simulink model "old_sync_block"  (R2015b)
settings: Solver=VariableStepAuto  StartTime=0.0  StopTime=10.0  RelTol=1e-3
undefined symbols (not defined in the file or in its folder): DiscIntNeverNeededParam, zh_step
libraries: simulink x2, dspnetwork x1
settings Model: Creator=Anony  LastModifiedBy=Anony

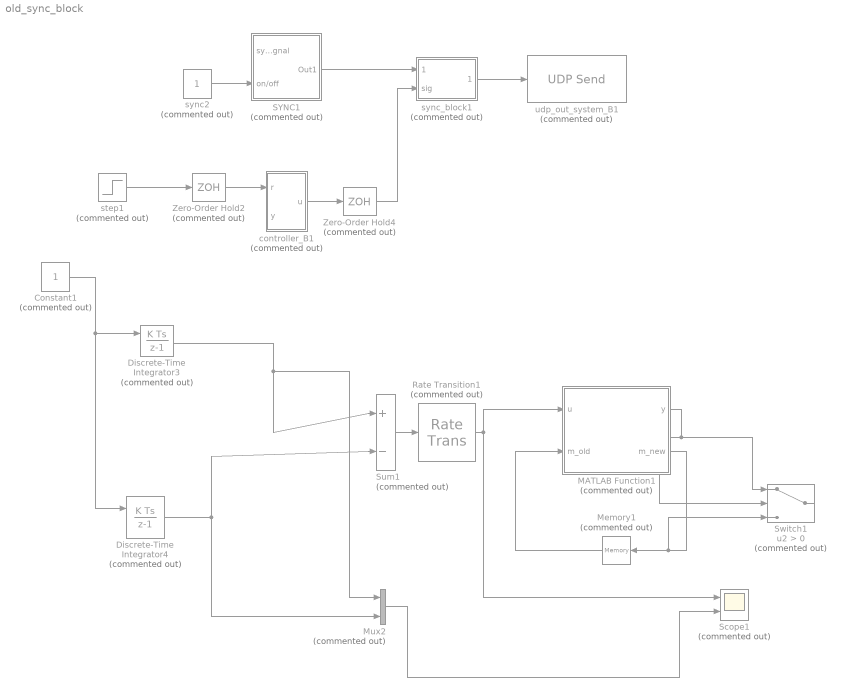
== system old_sync_block ==
  Constant1 : Constant  Commented=on
  Discrete-Time Integrator3 : DiscreteIntegrator  Commented=on  ExternalReset=rising  InitialConditionSetting=State (most efficient)  SampleTime=0.001  ICPrevOutput=DiscIntNeverNeededParam  ICPrevScaledInput=DiscIntNeverNeededParam
  Discrete-Time Integrator4 : DiscreteIntegrator  Commented=on  ExternalReset=rising  InitialConditionSetting=State (most efficient)  SampleTime=0.001  ICPrevOutput=DiscIntNeverNeededParam  ICPrevScaledInput=DiscIntNeverNeededParam
  MATLAB Function1 : MATLAB Function  Commented=on  TreatAsAtomicUnit=on
  Memory1 : Memory  Commented=on
  Mux2 : Mux  Commented=on  Inputs=2
  Rate Transition1 : RateTransition  Commented=on  OutPortSampleTimeOpt=Inherit
  SYNC1 : Subsystem  Commented=on
  Scope1 : Scope  Commented=on  NumInputPorts=2
  Sum1 : Sum  Commented=on  Inputs=|+-
  Switch1 : Switch  Commented=on  Criteria=u2 > Threshold
  Zero-Order Hold2 : ZeroOrderHold  Commented=on  SampleTime=zh_step
  Zero-Order Hold4 : ZeroOrderHold  Commented=on  SampleTime=zh_step
  controller_B1 : Subsystem  Commented=on
  step1 : Step  Commented=on  After=0.15  SampleTime=0
  sync2 : Constant  Commented=on
  sync_block1 : Subsystem  Commented=on
  udp_out_system_B1 : dspnetwork/UDP Send  Commented=on  remoteURL='129.10.131.51'  remotePort=27510  localURL='0.0.0.0'  localPortSource=Automatically determine  localPort=27000  sampletime=-1  separateLengthPort=0
  wires:
  step1/1 -> Zero-Order Hold2/1
  Zero-Order Hold2/1 -> controller_B1/1(r)
  controller_B1/1(u) -> Zero-Order Hold4/1
  sync_block1/1(sig out) -> udp_out_system_B1/1
  SYNC1/1(Out1) -> sync_block1/1(sync_sig)
  sync2/1 -> SYNC1/2(on/off)
  Zero-Order Hold4/1 -> sync_block1/2(sig)
  Discrete-Time Integrator3/1 -> Sum1/1, Mux2/1
  Constant1/1 -> Discrete-Time Integrator3/1, Discrete-Time Integrator4/1
  MATLAB Function1/2(m_new) -> Switch1/3, Memory1/1
  Sum1/1 -> Rate Transition1/1
  Memory1/1 -> MATLAB Function1/2(m_old)
  Discrete-Time Integrator4/1 -> Sum1/2, Mux2/2
  Mux2/1 -> Scope1/2
  MATLAB Function1/1(y) -> Switch1/1, Switch1/2
  Rate Transition1/1 -> MATLAB Function1/1(u), Scope1/1

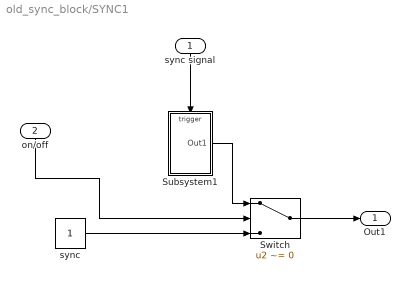
== system old_sync_block/SYNC1 ==
  sync signal : Inport
  on/off : Inport  Port=2
  Subsystem1 : Subsystem
  Switch : Switch  Criteria=u2 ~= 0
  sync : Constant
  Out1 : Outport
  wires:
  on/off/1 -> Switch/2
  Switch/1 -> Out1/1
  Subsystem1/1(Out1) -> Switch/1
  sync signal/1 -> Subsystem1/Trigger
  sync/1 -> Switch/3

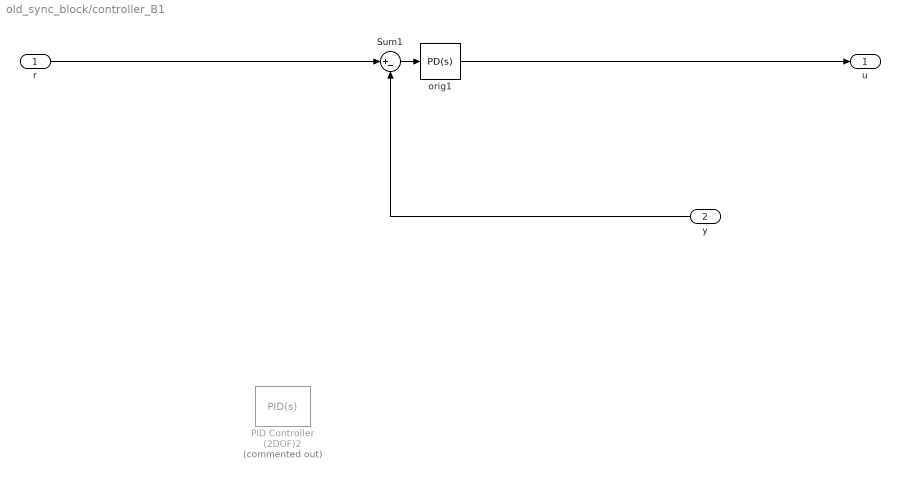
== system old_sync_block/controller_B1 ==
  r : Inport
  y : Inport  Port=2
  PID Controller (2DOF)2 : simulink/Continuous/PID Controller (2DOF)  Commented=on  Controller=PID  TimeDomain=Continuous-time  SampleTime=-1  IntegratorMethod=Forward Euler  FilterMethod=Forward Euler  Form=Parallel  UseFilter=on  ControllerParametersSource=internal  P=6.3799380872686  I=2.12979603411331  D=3.6093223618413  N=48.5068620404972  b=2.39624043732871  c=0.716079145801974  InitialConditionSource=internal  InitialConditionForIntegrator=0  InitialConditionForFilter=0  ExternalReset=none  LimitOutput=off  UpperSaturationLimit=inf  LowerSaturationLimit=-inf  LinearizeAsGain=on  AntiWindupMode=none  Kb=1  TrackingMode=off  Kt=1  PParamMin=[]  PParamMax=[]  IParamMin=[]  IParamMax=[]  DParamMin=[]  DParamMax=[]  NParamMin=[]  NParamMax=[]  bParamMin=[]  bParamMax=[]  cParamMin=[]  cParamMax=[]  KbParamMin=[]  KbParamMax=[]  KtParamMin=[]  KtParamMax=[]  POutMin=[]  POutMax=[]  IOutMin=[]  IOutMax=[]  DOutMin=[]  DOutMax=[]  NOutMin=[]  NOutMax=[]  bOutMin=[]  bOutMax=[]  cOutMin=[]  cOutMax=[]  KbOutMin=[]  KbOutMax=[]  KtOutMin=[]  KtOutMax=[]  IntegratorOutMin=[]  IntegratorOutMax=[]  FilterOutMin=[]  FilterOutMax=[]  SumOutMin=[]  SumOutMax=[]  Sum1OutMin=[]  Sum1OutMax=[]  Sum2OutMin=[]  Sum2OutMax=[]  Sum3OutMin=[]  Sum3OutMax=[]  SumI1OutMin=[]  SumI1OutMax=[]  SumI2OutMin=[]  SumI2OutMax=[]  SumI3OutMin=[]  SumI3OutMax=[]  SumDOutMin=[]  SumDOutMax=[]  SaturationOutMin=[]  SaturationOutMax=[]  IntegratorContinuousStateAttributes=''  IntegratorStateMustResolveToSignalObject=off  IntegratorRTWStateStorageClass=Auto  FilterContinuousStateAttributes=''  FilterStateMustResolveToSignalObject=off  FilterRTWStateStorageClass=Auto  DifferentiatorICPrevScaledInput=0  DifferentiatorOutMin=[]  DifferentiatorOutMax=[]
  Sum1 : Sum  Inputs=|+-
  orig1 : simulink/Continuous/PID Controller  Controller=PD  TimeDomain=Continuous-time  SampleTime=-1  IntegratorMethod=Forward Euler  FilterMethod=Forward Euler  Form=Parallel  UseFilter=on  ControllerParametersSource=internal  P=0.0142  I=0.0175856984919557  D=0.0001  N=100  InitialConditionSource=internal  InitialConditionForIntegrator=0  InitialConditionForFilter=0  ExternalReset=none  LimitOutput=on  UpperSaturationLimit=5/1000  LowerSaturationLimit=-5/1000  LinearizeAsGain=on  AntiWindupMode=none  Kb=1  TrackingMode=off  Kt=1  PParamMin=[]  PParamMax=[]  IParamMin=[]  IParamMax=[]  DParamMin=[]  DParamMax=[]  NParamMin=[]  NParamMax=[]  KbParamMin=[]  KbParamMax=[]  KtParamMin=[]  KtParamMax=[]  POutMin=[]  POutMax=[]  IOutMin=[]  IOutMax=[]  DOutMin=[]  DOutMax=[]  NOutMin=[]  NOutMax=[]  KbOutMin=[]  KbOutMax=[]  KtOutMin=[]  KtOutMax=[]  IntegratorOutMin=[]  IntegratorOutMax=[]  FilterOutMin=[]  FilterOutMax=[]  SumOutMin=[]  SumOutMax=[]  SumI1OutMin=[]  SumI1OutMax=[]  SumI2OutMin=[]  SumI2OutMax=[]  SumI3OutMin=[]  SumI3OutMax=[]  SumDOutMin=[]  SumDOutMax=[]  SaturationOutMin=[]  SaturationOutMax=[]  IntegratorContinuousStateAttributes=''  IntegratorStateMustResolveToSignalObject=off  IntegratorRTWStateStorageClass=Auto  FilterContinuousStateAttributes=''  FilterStateMustResolveToSignalObject=off  FilterRTWStateStorageClass=Auto  DifferentiatorICPrevScaledInput=0  DifferentiatorOutMin=[]  DifferentiatorOutMax=[]
  u : Outport
  wires:
  Sum1/1 -> orig1/1
  r/1 -> Sum1/1
  y/1 -> Sum1/2
  orig1/1 -> u/1

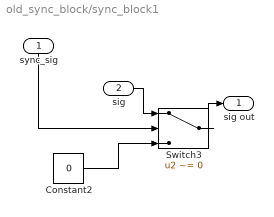
== system old_sync_block/sync_block1 ==
  sync_sig : Inport
  sig : Inport  Port=2
  Constant2 : Constant  Value=0
  Switch3 : Switch  Criteria=u2 ~= 0
  sig out : Outport
  wires:
  sync_sig/1 -> Switch3/2
  Switch3/1 -> sig out/1
  sig/1 -> Switch3/1
  Constant2/1 -> Switch3/3

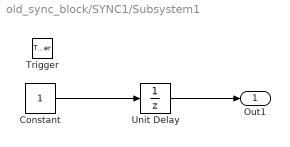
== system old_sync_block/SYNC1/Subsystem1 ==
  Trigger : TriggerPort  PortDimensions=1
  Constant : Constant
  Unit Delay : UnitDelay  SampleTime=-1
  Out1 : Outport
  wires:
  Constant/1 -> Unit Delay/1
  Unit Delay/1 -> Out1/1

== matlab function old_sync_block/MATLAB Function1 ==
  data: u input; y output; m_new output; m_old input
function [y,m_new] = fcn(u,m_old)
%#codegen
if(u>0)
    y = u;
    m_new = u;
else
    y =0;
    m_new = m_old;
end
